simulink model "test_SOC"  (R2024a)
settings: Solver=FixedStepAuto  StartTime=0.0  StopTime=stop_time  FixedStep=Ts  RelTol=1e-3
settings Model: Creator=mmackenzie  LastModifiedBy=mmackenzie

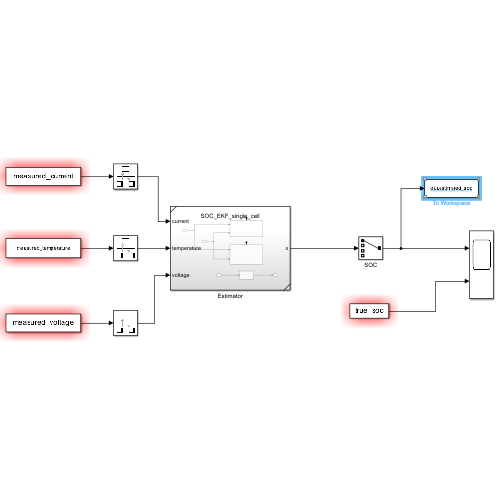
[thumbnail: Simulink's stored preview of the top-level diagram]
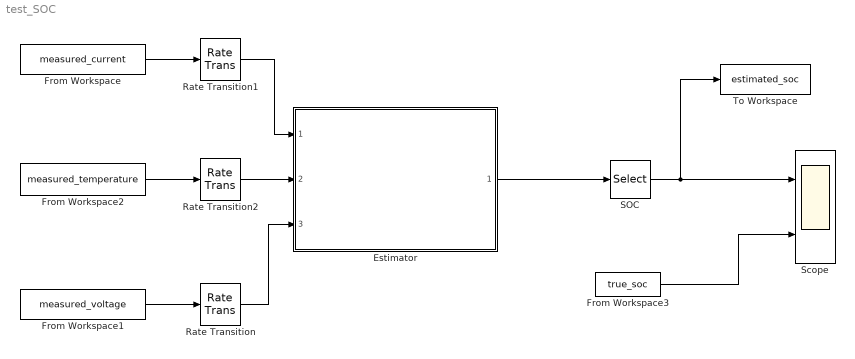
== system test_SOC ==
  Estimator : Subsystem  ReferencedSubsystem=SOC_EKF_single_cell
      settings: PermitHierarchicalResolution=None
  From Workspace : FromWorkspace  VariableName=measured_current
  From Workspace1 : FromWorkspace  VariableName=measured_voltage
  From Workspace2 : FromWorkspace  VariableName=measured_temperature
  From Workspace3 : FromWorkspace  VariableName=true_soc
  Rate Transition : RateTransition
  Rate Transition1 : RateTransition
  Rate Transition2 : RateTransition
  SOC : Selector  InputPortWidth=4  IndexOptions=Index vector (dialog)  Indices=1  OutputSizes=1
  Scope : Scope  NumInputPorts=2
  To Workspace : ToWorkspace  VariableName=estimated_soc  SaveFormat=Timeseries  SampleTime=-1
  wires:
  Estimator/1 -> SOC/1
  SOC/1 -> To Workspace/1, Scope/1
  From Workspace/1 -> Rate Transition1/1
  From Workspace2/1 -> Rate Transition2/1
  From Workspace1/1 -> Rate Transition/1
  From Workspace3/1 -> Scope/2
  Rate Transition/1 -> Estimator/3
  Rate Transition1/1 -> Estimator/1
  Rate Transition2/1 -> Estimator/2
